simulink library "TB_blk_library"  (R2019b)
settings: Solver=VariableStepAuto  StartTime=0.0  StopTime=10.0  RelTol=1e-3
undefined symbols (not defined in the file or in its folder): maxF
settings Model: Creator=gurtnmar  LastModifiedBy=gurtnmar
settings DataIOCC: ReturnWorkspaceOutputs=off
settings DebuggingCC: ArithmeticOperatorsInVariantConditions=warning
settings SFSimCC: SimUseLocalCustomCode=off  CustomCodeUndefinedFunction=UseInterfaceOnly
settings RTWCC: RTWUseLocalCustomCode=off
settings CodeAppCC: StateflowObjectComments=on

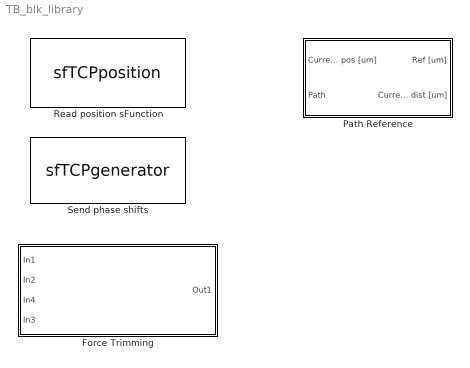
== system TB_blk_library ==
  Force Trimming : Subsystem  mask{maxFstruct=maxF}
      mask prompts: maxFstruct "Fmax structure"
      mask Display:
      | disp('8-way force trimming')
      | port_label('input',  1, '[Fx;Fy;Fz]')
      | port_label('input',  2, '[x;y;z]')
      | port_label('input',  3, '8-dir flag')
      | port_label('input',  4, 'maxForce flag')
      | port_label('output', 1, '[Fx;Fy;Fz]')
  Path Reference : Subsystem  mask{switch_dist=20, repeat=off}
      mask prompts: switch_dist "Switching distance [um]"
  Read position sFunction : S-Function  FunctionName=sfTCPposition  Parameters=Ts,ip_addr,tcp_port,N_objs,track_in_RG  SFunctionDeploymentMode=off  EnableBusSupport=off  mask{Ts=1/30, ip_addr='147.32.86.138', tcp_port=30000, N_objs=2, track_in_RG=on}
      mask prompts: Ts "Sampling period"; ip_addr "IP address"; tcp_port "TCP port"; N_objs "Number of objects"; track_in_RG "Track in both color channels"
      mask Display:
      | ipaddr = get_param(gcb,'ip_addr');
      | port = get_param(gcb,'tcp_port');
      | % disp('Read Position (TCP)')
      | fprintf('Read Position (TCP)\n IP:%s \n port: %s', ipaddr, port);
  Send phase shifts : S-Function  FunctionName=sfTCPgenerator  Parameters=Ts,ip_addr,tcp_port  SFunctionDeploymentMode=off  EnableBusSupport=off  mask{Ts=1/30, ip_addr='147.32.86.138', tcp_port=30001}
      mask prompts: Ts "Sampling period"; ip_addr "IP address"; tcp_port "TCP port"
      mask Display:
      | ipaddr = get_param(gcb,'ip_addr');
      | port = get_param(gcb,'tcp_port');
      | fprintf('Generator (TCP)\n IP:%s \n port: %s', ipaddr, port);

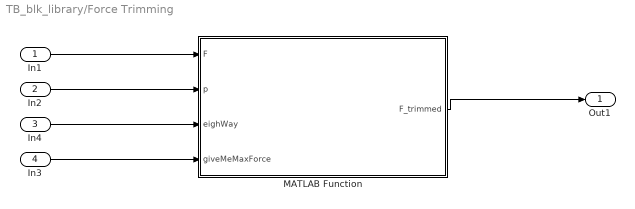
== system TB_blk_library/Force Trimming ==
  In1 : Inport
  In2 : Inport  Port=2
  In4 : Inport  Port=3
  In3 : Inport  Port=4
  MATLAB Function : MATLAB Function  TreatAsAtomicUnit=on
  Out1 : Outport
  wires:
  MATLAB Function/1(F_trimmed) -> Out1/1
  In1/1 -> MATLAB Function/1(F)
  In2/1 -> MATLAB Function/2(p)
  In3/1 -> MATLAB Function/4(giveMeMaxForce)
  In4/1 -> MATLAB Function/3(eighWay)

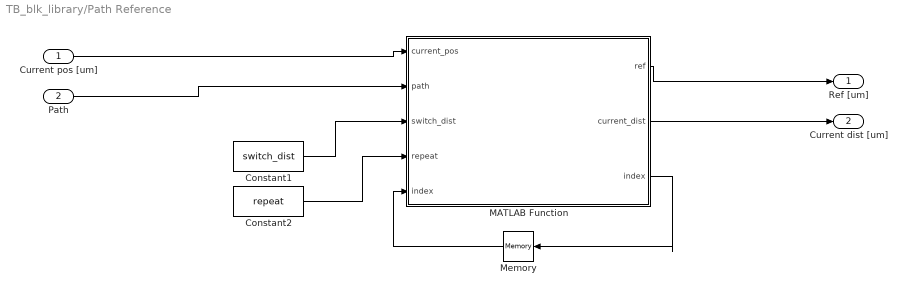
== system TB_blk_library/Path Reference ==
  Current pos [um] : Inport
  Path : Inport  Port=2
  Constant1 : Constant  Value=switch_dist
  Constant2 : Constant  Value=repeat
  MATLAB Function : MATLAB Function  TreatAsAtomicUnit=on
  Memory : Memory  InitialCondition=1
  Ref [um] : Outport
  Current dist [um] : Outport  Port=2
  wires:
  Constant1/1 -> MATLAB Function/3(switch_dist)
  Constant2/1 -> MATLAB Function/4(repeat)
  MATLAB Function/3(index) -> Memory/1
  MATLAB Function/1(ref) -> Ref [um]/1
  Current pos [um]/1 -> MATLAB Function/1(current_pos)
  Memory/1 -> MATLAB Function/5("index ")
  Path/1 -> MATLAB Function/2(path)
  MATLAB Function/2(current_dist) -> Current dist [um]/1

== matlab function TB_blk_library/Path Reference/MATLAB Function ==
  data: current_pos input; path input; switch_dist input; repeat input; ref output; current_dist output; index input; index output
function [ref, current_dist, index] = fcn(current_pos, path, switch_dist, repeat, index)
% path = [x0 ... xn; y0 ... yn]
% current_pos = [x; y]

current_dist = sqrt((path(1, index) - current_pos(1))^2 + (path(2, index) - current_pos(2))^2);

if current_dist < switch_dist
    index = index + 1;
end

if index > size(path, 2)
    if repeat
        index = 1;
    else
        index = size(path, 2);
    end
end

ref = path(1:2, index);

== matlab function TB_blk_library/Force Trimming/MATLAB Function ==
  data: F input; F_trimmed output; p input; maxFstruct parameter; eighWay input; giveMeMaxForce input
function F_trimmed = fcn(F, p, maxFstruct, eighWay, giveMeMaxForce)
    F_trimmed = F;
    if eighWay
        F_trimmed(1:2) = clipTheForce_nearest(F(1:2), p(1), p(2), maxFstruct, giveMeMaxForce);
    else
        F_trimmed(1:2) = clipTheForce(F(1:2), p(1), p(2), maxFstruct, giveMeMaxForce);
    end
end
